simulink model "Linear_Moving_Setpoint"  (R2020b)
settings: Solver=VariableStepAuto  StartTime=0.0  StopTime=t_sim  RelTol=1e-9
undefined symbols (not defined in the file): A1_sim, B1_sim, C1_setp_ctrl, den1, K1, KI, KP, omega_sim, Plant_Inv_TF, r_sim, SP_sel, x1_0
libraries: simulink x1
settings Model: Creator=domin  LastModifiedBy=domin

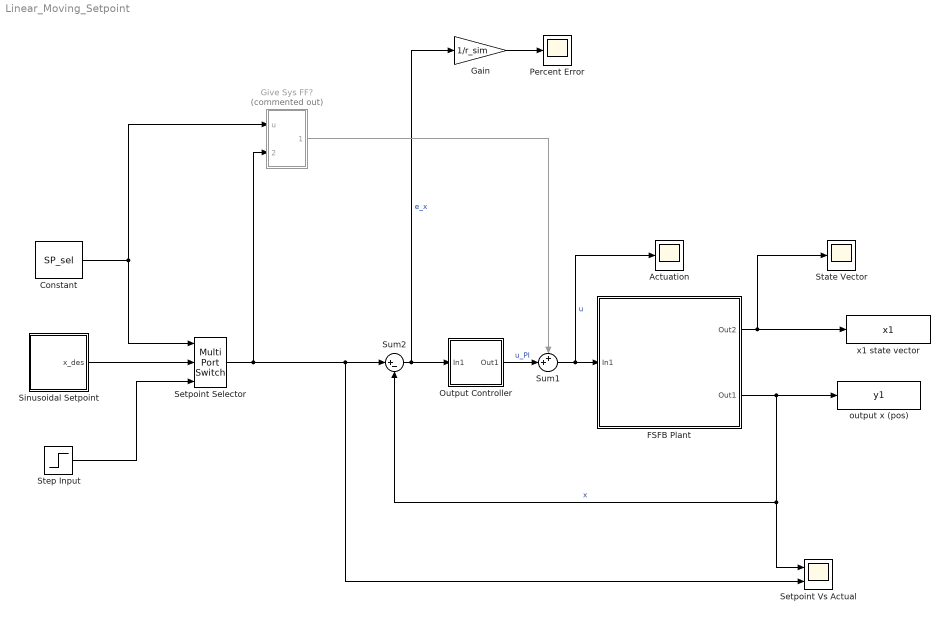
== system Linear_Moving_Setpoint ==
  Actuation : Scope
  Constant : Constant  Value=SP_sel
  FSFB Plant : Subsystem
  Gain : Gain  Gain=1/r_sim
  Give Sys FF? : Subsystem  Commented=on
  Output Controller : Subsystem
  Percent Error : Scope
  Setpoint Selector : MultiPortSwitch  Inputs=2
  Setpoint Vs Actual : Scope  NumInputPorts=2
  Sinusoidal Setpoint : Subsystem
  State Vector : Scope
  Step Input : Step  After=r_sim  SampleTime=0
  Sum1 : Sum  Inputs=++|
  Sum2 : Sum  Inputs=|+-
  output x (pos) : ToWorkspace  VariableName=y1  SampleTime=-1
  x1 state vector : ToWorkspace  VariableName=x1  SampleTime=-1
  wires:
  Sum2/1 -> Output Controller/1(In1), Gain/1  "e_x"
  FSFB Plant/2(Out1) -> Sum2/2, Setpoint Vs Actual/1, output x (pos)/1  "x"
  Output Controller/1(Out1) -> Sum1/2  "u_PI"
  FSFB Plant/1(Out2) -> x1 state vector/1, State Vector/1
  Gain/1 -> Percent Error/1
  Setpoint Selector/1 -> Give Sys FF?/2(In2), Setpoint Vs Actual/2, Sum2/1
  Sinusoidal Setpoint/1(x_des) -> Setpoint Selector/2
  Step Input/1 -> Setpoint Selector/3
  Constant/1 -> Setpoint Selector/1, Give Sys FF?/1(u)
  Sum1/1 -> Actuation/1, FSFB Plant/1(In1)  "u"
  Give Sys FF?/1(Out1) -> Sum1/1

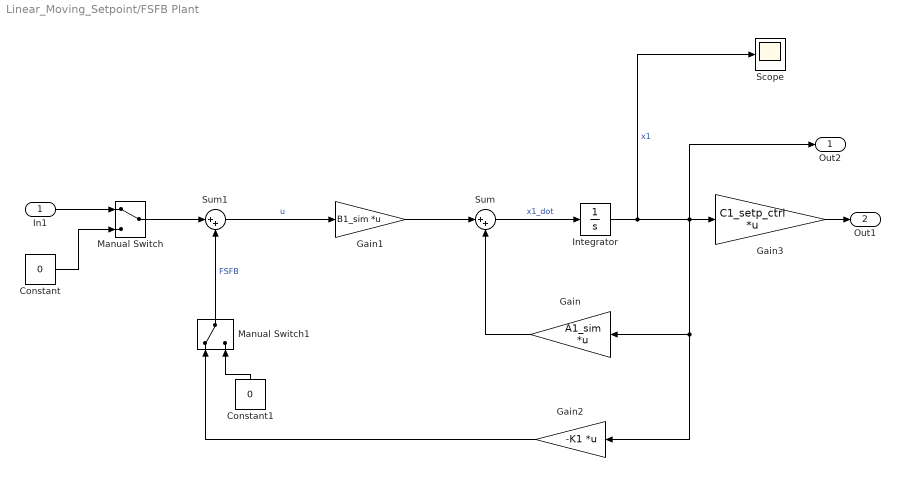
== system Linear_Moving_Setpoint/FSFB Plant ==
  In1 : Inport
  Constant : Constant  Value=0
  Constant1 : Constant  Value=0
  Gain : Gain  Gain=A1_sim  Multiplication=Matrix(K*u)
  Gain1 : Gain  Gain=B1_sim  Multiplication=Matrix(K*u)
  Gain2 : Gain  Gain=-K1  Multiplication=Matrix(K*u)
  Gain3 : Gain  Gain=C1_setp_ctrl  Multiplication=Matrix(K*u)
  Integrator : Integrator  InitialCondition=x1_0
  Manual Switch : ManualSwitch
  Manual Switch1 : ManualSwitch
  Scope : Scope
  Sum : Sum  Inputs=|++
  Sum1 : Sum  Inputs=|++
  Out2 : Outport
  Out1 : Outport  Port=2
  wires:
  Gain1/1 -> Sum/1
  Sum/1 -> Integrator/1  "x1_dot"
  Integrator/1 -> Scope/1, Out2/1, Gain2/1, Gain/1, Gain3/1  "x1"
  Gain3/1 -> Out1/1
  Gain/1 -> Sum/2
  In1/1 -> Manual Switch/1
  Constant/1 -> Manual Switch/2
  Sum1/1 -> Gain1/1  "u"
  Gain2/1 -> Manual Switch1/1
  Manual Switch/1 -> Sum1/1
  Manual Switch1/1 -> Sum1/2  "FSFB"
  Constant1/1 -> Manual Switch1/2

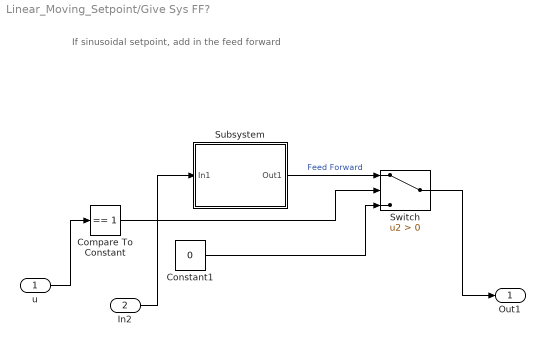
== system Linear_Moving_Setpoint/Give Sys FF? ==
  note: If sinusoidal setpoint, add in the feed forward
  u : Inport
  In2 : Inport  Port=2
  Compare To Constant : simulink/Logic and Bit Operations/Compare To Constant  relop===  const=1  OutDataTypeStr=boolean
  Constant1 : Constant  Value=0
  Subsystem : Subsystem
  Switch : Switch  Criteria=u2 > Threshold
  Out1 : Outport
  wires:
  Switch/1 -> Out1/1
  u/1 -> Compare To Constant/1
  Subsystem/1(Out1) -> Switch/1  "Feed Forward"
  Compare To Constant/1 -> Switch/2
  Constant1/1 -> Switch/3
  In2/1 -> Subsystem/1(In1)

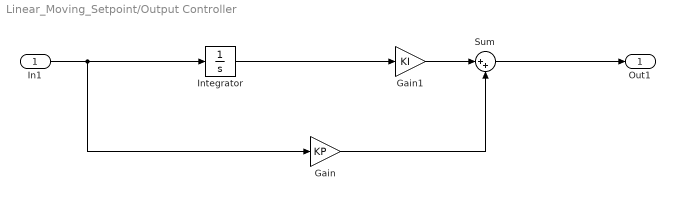
== system Linear_Moving_Setpoint/Output Controller ==
  In1 : Inport
  Gain : Gain  Gain=KP
  Gain1 : Gain  Gain=KI
  Integrator : Integrator
  Sum : Sum  Inputs=|++
  Out1 : Outport
  wires:
  In1/1 -> Integrator/1, Gain/1
  Gain/1 -> Sum/2
  Gain1/1 -> Sum/1
  Sum/1 -> Out1/1
  Integrator/1 -> Gain1/1

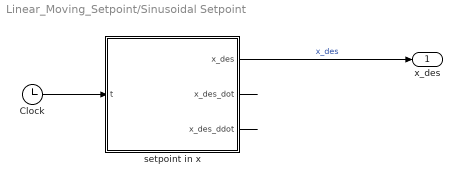
== system Linear_Moving_Setpoint/Sinusoidal Setpoint ==
  Clock : Clock
  setpoint in x : MATLAB Function  TreatAsAtomicUnit=on
  x_des : Outport
  wires:
  Clock/1 -> setpoint in x/1(t)
  setpoint in x/3(x_des_ddot) -> ?
  setpoint in x/2(x_des_dot) -> ?
  setpoint in x/1(x_des) -> x_des/1  "x_des"

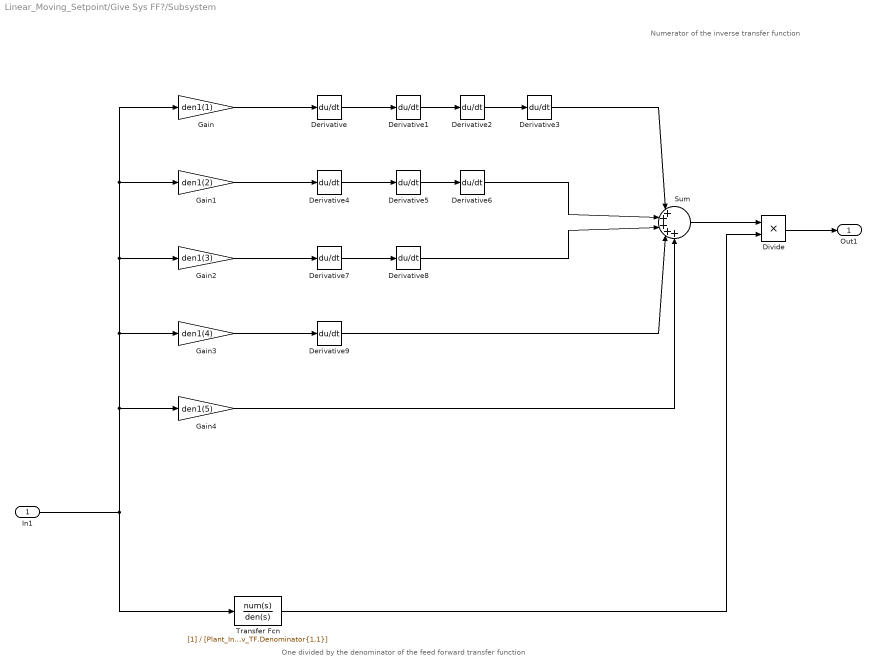
== system Linear_Moving_Setpoint/Give Sys FF?/Subsystem ==
  note: Numerator of the inverse transfer function
  note: One divided by the denominator of the feed forward transfer function
  In1 : Inport
  Derivative{,1..9} (10 alike) : Derivative
  Divide : Product  Inputs=**
  Gain : Gain  Gain=den1(1)
  Gain1 : Gain  Gain=den1(2)
  Gain2 : Gain  Gain=den1(3)
  Gain3 : Gain  Gain=den1(4)
  Gain4 : Gain  Gain=den1(5)
  Sum : Sum  Inputs=|+++++
  Transfer Fcn : TransferFcn  Denominator=[Plant_Inv_TF.Denominator{1,1}]
  Out1 : Outport
  wires:
  Gain/1 -> Derivative/1
  Derivative/1 -> Derivative1/1
  Derivative1/1 -> Derivative2/1
  Derivative2/1 -> Derivative3/1
  In1/1 -> Transfer Fcn/1, Gain1/1, Gain/1, Gain2/1, Gain3/1, Gain4/1
  Derivative5/1 -> Derivative6/1
  Derivative4/1 -> Derivative5/1
  Gain1/1 -> Derivative4/1
  Gain2/1 -> Derivative7/1
  Derivative7/1 -> Derivative8/1
  Gain3/1 -> Derivative9/1
  Derivative3/1 -> Sum/1
  Derivative6/1 -> Sum/2
  Derivative8/1 -> Sum/3
  Derivative9/1 -> Sum/4
  Gain4/1 -> Sum/5
  Sum/1 -> Divide/1
  Transfer Fcn/1 -> Divide/2
  Divide/1 -> Out1/1

== matlab function Linear_Moving_Setpoint/Sinusoidal Setpoint/setpoint in x ==
  data: t input; x_des output; x_des_dot output; x_des_ddot output; r_sim parameter; omega_sim parameter
function [x_des,x_des_dot,x_des_ddot] = fcn(t,r_sim, omega_sim)

w = omega_sim;
r = r_sim;

x_des = r*sin(w*t);
x_des_dot = r*w*cos(w*t);
x_des_ddot = -r*w^2*sin(w*t);
